simulink model "ex_3s0"  (R2018b)
settings: Solver=ode5  StartTime=0.0  StopTime=45  FixedStep=0.001  RelTol=1e-3
libraries: discretizing x1
settings Model: Creator=lenovo  LastModifiedBy=QJ-
settings DebuggingCC: LibraryContextMissingDiagnostic=none
settings SFSimCC: SimUseLocalCustomCode=off
settings RTWCC: RTWUseLocalCustomCode=off

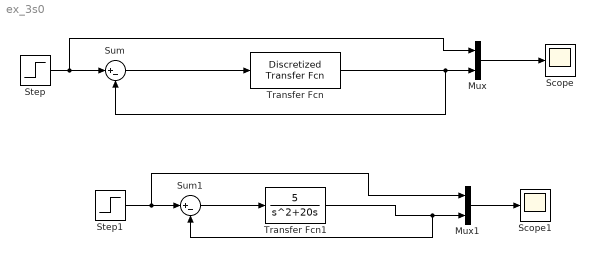
== system ex_3s0 ==
  Mux : Mux  Inputs=2
  Mux1 : Mux  Inputs=2
  Scope : Scope
  Scope1 : Scope
  Step : Step  SampleTime=1  mask(DiscretizedSource){}
      mask init:
      | %zoh
  Step1 : Step  SampleTime=1  mask(DiscretizedSource){}
      mask init:
      | %zoh
  Sum : Sum  Inputs=|+-
  Sum1 : Sum  Inputs=|+-
  Transfer Fcn : discretizing/Discretized Transfer Fcn  Numerator=[5]  Denominator=[1 20 0]  AbsTol=auto  SampleTime=0.001  method=zoh  Wc=1
  Transfer Fcn1 : TransferFcn  Numerator=[5]  Denominator=[1 20 0]
  wires:
  Transfer Fcn/1 -> Sum/2, Mux/2
  Sum/1 -> Transfer Fcn/1
  Step/1 -> Mux/1, Sum/1
  Mux/1 -> Scope/1
  Sum1/1 -> Transfer Fcn1/1
  Step1/1 -> Mux1/1, Sum1/1
  Transfer Fcn1/1 -> Sum1/2, Mux1/2
  Mux1/1 -> Scope1/1
